simulink model "MotorTests"  (R2023b)
settings: Solver=VariableStepAuto  StartTime=0.0  StopTime=10.0  RelTol=1e-3
libraries: spsCurrentMeasurementLib x4, spsVoltageMeasurementLib x4, spsGroundLib x3, spsAsynchronousMachineSIUnitsLib x2, spsRMSLib x2, spspowerguiLib x2, mcbacimparamestlib x2, spsDCVoltageSourceLib x1, spsPowerPositiveSequenceLib x1, spsThreePhaseProgrammableVoltageSourceLib x1
settings Model: Creator=Jakob  LastModifiedBy=Jakob

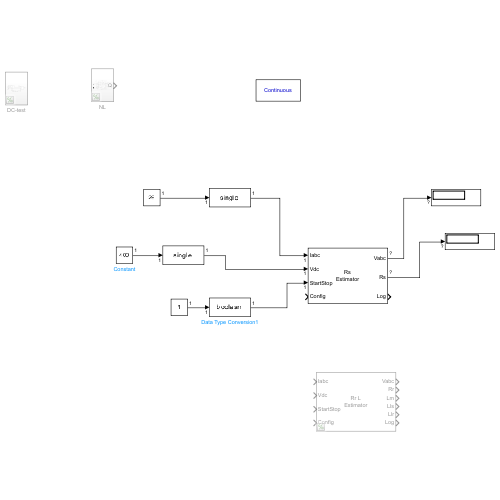
[thumbnail: Simulink's stored preview of the top-level diagram]
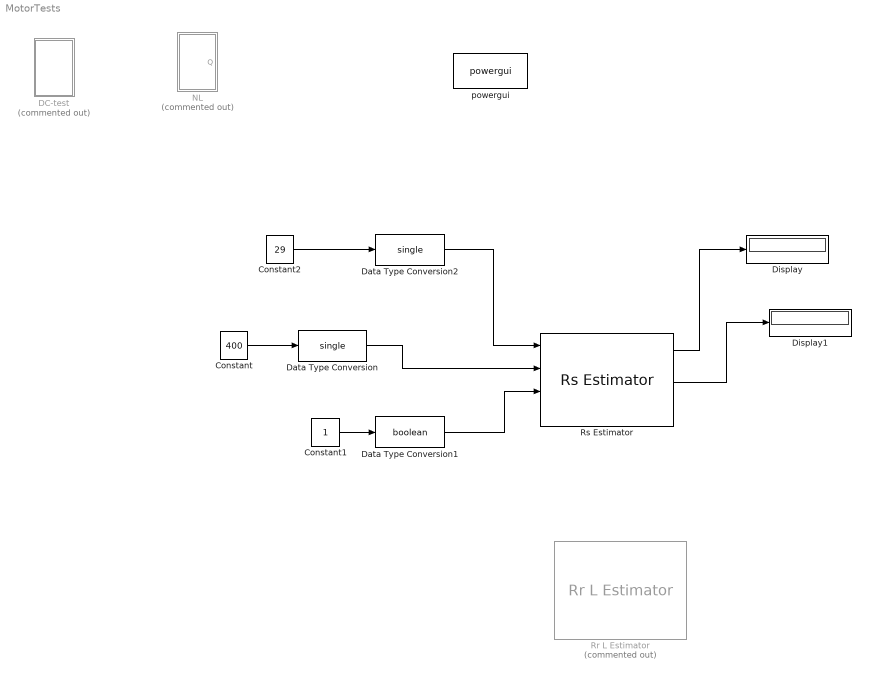
== system MotorTests ==
  Constant : Constant  Value=400
  Constant1 : Constant
  Constant2 : Constant  Value=29
  DC-test : Subsystem  Commented=on
  Data Type Conversion : DataTypeConversion  OutDataTypeStr=single  SaturateOnIntegerOverflow=off  RndMeth=Floor
  Data Type Conversion1 : DataTypeConversion  OutDataTypeStr=boolean  SaturateOnIntegerOverflow=off  RndMeth=Floor
  Data Type Conversion2 : DataTypeConversion  OutDataTypeStr=single  SaturateOnIntegerOverflow=off  RndMeth=Floor
  Display : Display
  Display1 : Display
  NL : Subsystem  Commented=on
  Rr L Estimator : mcbacimparamestlib/Rr L Estimator  Commented=on
      settings: LibrarySourceBlock=mcblib/Parameter Estimation/ACIM Parameter Estimation/Rr L Estimator
  Rs Estimator : mcbacimparamestlib/Rs Estimator
      settings: LibrarySourceBlock=mcblib/Parameter Estimation/ACIM Parameter Estimation/Rs Estimator
  powergui : spspowerguiLib/powergui  Priority=1  SimulationMode=Continuous  SampleTime=50e-6  frequency=60  Iterations=50  frequencyindice=50  Pbase=100e6  ErrMax=1e-4  UnitsV=kV  UnitsW=MW  buscounter=0  FunctionMessages=off  echomessages=off  EnableUseOfTLC=off  CurrentSourceSwitches=off  DisableSnubberDevices=off  DisableRonSwitches=off  DisableVfSwitches=off  DisplayEquations=off  AutomaticDiscreteSolvers=off  SolverType=Tustin/Backward Euler (TBE)  Interpol=off  ExternalGateDelay=off  methode=off  Ts=100  x0status=blocks  SPID=on  SwTol=0  HookPort=off  NonlinearTolerance=1e-4  nMaxIteration=100  ContinueOnMaxIteration=off  RestoreLinks=warning  ResistiveCurrentMeasurement=off  Frange=[0:2:500]  Ylog=off  Xlog=on  ShowGrid=off  save=off  variable=ZData  structure=0  ZoomFFT=off  StartTime=0.0  cycles=1  DisplayStyle=1  fundamental=60  FreqAxis=off  MaxFrequency=1000  frequencyindicesteady=1  RmsSteady=1  display=off
  wires:
  Constant/1 -> Data Type Conversion/1
  Constant1/1 -> Data Type Conversion1/1
  Rs Estimator/1 -> Display/1
  Rs Estimator/2 -> Display1/1
  Data Type Conversion/1 -> Rs Estimator/2
  Data Type Conversion1/1 -> Rs Estimator/3
  Constant2/1 -> Data Type Conversion2/1
  Data Type Conversion2/1 -> Rs Estimator/1

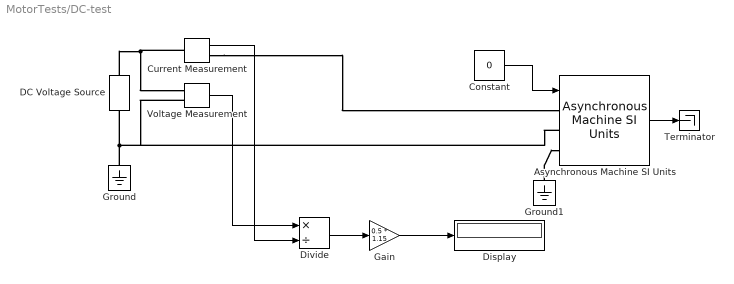
== system MotorTests/DC-test ==
  Asynchronous Machine SI Units : spsAsynchronousMachineSIUnitsLib/Asynchronous Machine SI Units  RotorType=Double squirrel-cage  PresetModel=No  MechanicalLoad=Torque Tm  ShowDetailedParameters=on  ReferenceFrame=Rotor  Units=SI  MeasurementBus=off  NominalParameters=[1.5e+04 400 50]  VoltageRatio=1  Stator=[0.619 0.0005084]  Rotor=[0.6258 0.005473]  Cage1=[0.2781 0.002617]  Cage2=[0.5433 0.0005084]  Lm=0.04417  Mechanical=[0.13 0.005879 2]  PolePairs=2  InitialConditions=[0 0 0 0 0 0 0 0]  SimulateSaturation=off  Saturation=[14.03593122, 27.81365428, 53.79336849, 72.68890987, 97.98006896, 148.6815601, 215.7428561, 302.9841135, 428.7778367 ; 230, 322, 414, 460, 506, 552, 598, 644, 690]  LoadFlowParameters=1492000  TsPowergui=0  TsBlock=-1  IterativeModel=Trapezoidal non iterative  IterativeDiscreteModel=Trapezoidal non iterative  Pmec=1.492e+006
  Constant : Constant  Value=0
  Current Measurement : spsCurrentMeasurementLib/Current Measurement  PhasorSimulation=off  OutputType=Complex  PSBequivalent=0
  DC Voltage Source : spsDCVoltageSourceLib/DC Voltage Source  Amplitude=9  Measurements=None
  Display : Display
  Divide : Product  Inputs=*/
  Gain : Gain  Gain=0.5 * 1.15
  Ground : spsGroundLib/Ground  LConnTagsString=a
  Ground1 : spsGroundLib/Ground  LConnTagsString=a
  Terminator : Terminator
  Voltage Measurement : spsVoltageMeasurementLib/Voltage Measurement  PhasorSimulation=off  OutputType=Complex  PSBequivalent=0
  wires:
  Constant/1 -> Asynchronous Machine SI Units/1
  Voltage Measurement/1 -> Divide/1
  Divide/1 -> Gain/1
  Asynchronous Machine SI Units/1 -> Terminator/1
  Gain/1 -> Display/1
  Current Measurement/1 -> Divide/2
  connections:
  Ground1/LConn1 -- Asynchronous Machine SI Units/LConn3
  DC Voltage Source/RConn1 -- Voltage Measurement/LConn1 -- Current Measurement/LConn1
  Ground/LConn1 -- Asynchronous Machine SI Units/LConn2 -- Voltage Measurement/LConn2 -- DC Voltage Source/LConn1
  Current Measurement/RConn1 -- Asynchronous Machine SI Units/LConn1

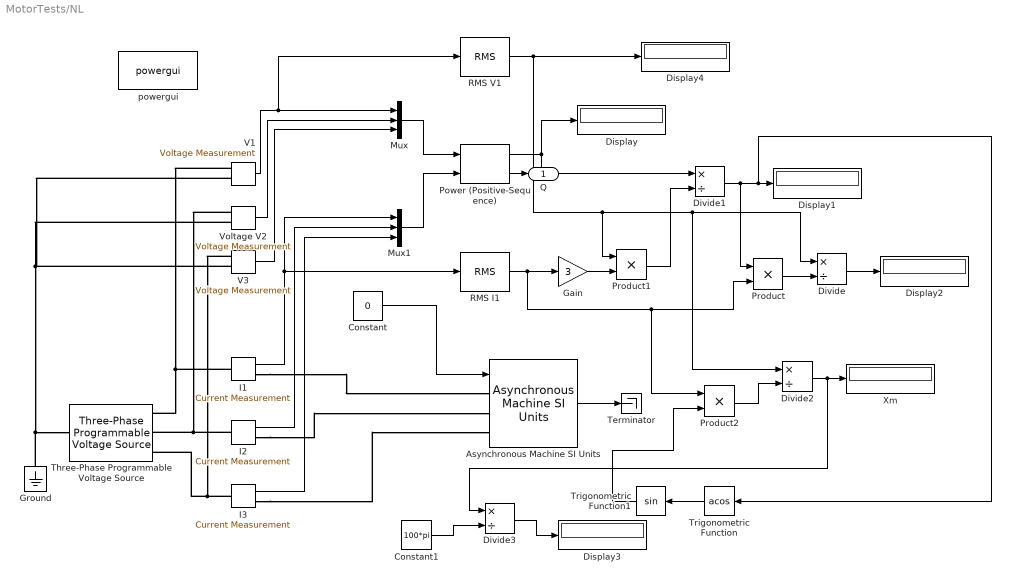
== system MotorTests/NL ==
  Asynchronous Machine SI Units : spsAsynchronousMachineSIUnitsLib/Asynchronous Machine SI Units  RotorType=Double squirrel-cage  PresetModel=No  MechanicalLoad=Torque Tm  ShowDetailedParameters=on  ReferenceFrame=Rotor  Units=SI  MeasurementBus=off  NominalParameters=[1.5e+04 400 50]  VoltageRatio=1  Stator=[0.619 0.0005084]  Rotor=[0.6258 0.005473]  Cage1=[0.2781 0.002617]  Cage2=[0.5433 0.0005084]  Lm=0.04417  Mechanical=[0.13 0.005879 2]  PolePairs=2  InitialConditions=[1 0 0 0 0 0 0 0]  SimulateSaturation=off  Saturation=[14.03593122, 27.81365428, 53.79336849, 72.68890987, 97.98006896, 148.6815601, 215.7428561, 302.9841135, 428.7778367 ; 230, 322, 414, 460, 506, 552, 598, 644, 690]  LoadFlowParameters=1492000  TsPowergui=0  TsBlock=-1  IterativeModel=Trapezoidal non iterative  IterativeDiscreteModel=Trapezoidal non iterative  Pmec=1.492e+006
  Constant : Constant  Value=0
  Constant1 : Constant  Value=100*pi
  Display{,1..4} (5 alike) : Display
  Divide{,1..3} (4 alike) : Product  Inputs=*/
  Gain : Gain  Gain=3
  Ground : spsGroundLib/Ground  LConnTagsString=a
  I1 : spsCurrentMeasurementLib/Current Measurement  PhasorSimulation=off  OutputType=Complex  PSBequivalent=0
  I2 : spsCurrentMeasurementLib/Current Measurement  PhasorSimulation=off  OutputType=Complex  PSBequivalent=0
  I3 : spsCurrentMeasurementLib/Current Measurement  PhasorSimulation=off  OutputType=Complex  PSBequivalent=0
  Mux : Mux  Inputs=3
  Mux1 : Mux  Inputs=3
  Power (Positive-Sequence) : spsPowerPositiveSequenceLib/Power (Positive-Sequence)  Freq=60  Vinit=[0, 0]  Iinit=[0, 0]  Ts=0
      settings: LibrarySourceBlock=|
      | sps_lib/Sensors and Measurements/Power
      | (Positive-Sequence)
  Product : Product
  Product1 : Product
  Product2 : Product
  RMS I1 : spsRMSLib/RMS  TrueRMS=on  Freq=60  RMSInit=120  Ts=0
  RMS V1 : spsRMSLib/RMS  TrueRMS=on  Freq=60  RMSInit=120  Ts=0
  Terminator : Terminator
  Three-Phase Programmable Voltage Source : spsThreePhaseProgrammableVoltageSourceLib/Three-Phase Programmable Voltage Source  PositiveSequence="[400  0 50]"  VariationEntity=None  VariationType=Table of time-amplitude pairs  VariationTypeAlt=Step  VariationStep=0.5  VariationRate=10  VariationMagnitude=0.3  VariationFrequency=2  VariationTiming=[1 2]  VariationPhaseA=off  Amplitudes=[1 0.8 1.2 1.0]  TimeValues=[0 0.1 0.15 0.2]  HarmonicGeneration=off  HarmonicA=[3 0.2 -25 0]  HarmonicB=[2 0.15 35 2]  Timing="[0.05  3]"  BusType=swing  Pref=0  Qref=0  Qmin=-inf  Qmax=inf
  Trigonometric Function : Trigonometry  Operator=acos
  Trigonometric Function1 : Trigonometry
  V1 : spsVoltageMeasurementLib/Voltage Measurement  PhasorSimulation=off  OutputType=Complex  PSBequivalent=0
  V3 : spsVoltageMeasurementLib/Voltage Measurement  PhasorSimulation=off  OutputType=Complex  PSBequivalent=0
  Voltage V2 : spsVoltageMeasurementLib/Voltage Measurement  PhasorSimulation=off  OutputType=Complex  PSBequivalent=0
  Xm : Display
  powergui : spspowerguiLib/powergui  Priority=1  SimulationMode=Continuous  SampleTime=50e-6  frequency=60  Iterations=50  frequencyindice=50  Pbase=100e6  ErrMax=1e-4  UnitsV=kV  UnitsW=MW  buscounter=0  FunctionMessages=off  echomessages=off  EnableUseOfTLC=off  CurrentSourceSwitches=off  DisableSnubberDevices=off  DisableRonSwitches=off  DisableVfSwitches=off  DisplayEquations=off  AutomaticDiscreteSolvers=off  SolverType=Tustin/Backward Euler (TBE)  Interpol=off  ExternalGateDelay=off  methode=off  Ts=100  x0status=blocks  SPID=on  SwTol=0  HookPort=off  NonlinearTolerance=1e-4  nMaxIteration=100  ContinueOnMaxIteration=off  RestoreLinks=warning  ResistiveCurrentMeasurement=off  Frange=[0:2:500]  Ylog=off  Xlog=on  ShowGrid=off  save=off  variable=ZData  structure=0  ZoomFFT=off  StartTime=0.0  cycles=1  DisplayStyle=1  fundamental=60  FreqAxis=off  MaxFrequency=1000  frequencyindicesteady=1  RmsSteady=1  display=off
  Q : Outport
  wires:
  RMS V1/1 -> Display4/1, Divide2/1, Divide/1, Product1/1
  Constant1/1 -> Divide3/2
  I1/1 -> RMS I1/1, Mux1/1
  Divide/1 -> Display2/1
  Mux1/1 -> Power (Positive-Sequence)/2
  V1/1 -> RMS V1/1, Mux/1
  I3/1 -> Mux1/3
  Power (Positive-Sequence)/1 -> Divide1/1, Display/1
  Constant/1 -> Asynchronous Machine SI Units/1
  Mux/1 -> Power (Positive-Sequence)/1
  RMS I1/1 -> Product2/1, Product/2, Gain/1
  Product/1 -> Divide/2
  Divide2/1 -> Divide3/1, Xm/1
  Asynchronous Machine SI Units/1 -> Terminator/1
  Divide1/1 -> Product/1, Display1/1, Trigonometric Function/1
  Trigonometric Function/1 -> Trigonometric Function1/1
  Gain/1 -> Product1/2
  Product1/1 -> Divide1/2
  Power (Positive-Sequence)/2 -> Q/1
  Voltage V2/1 -> Mux/2
  Product2/1 -> Divide2/2
  V3/1 -> Mux/3
  I2/1 -> Mux1/2
  Trigonometric Function1/1 -> Product2/2
  Divide3/1 -> Display3/1
  connections:
  I3/LConn1 -- V3/LConn1 -- Three-Phase Programmable Voltage Source/RConn3
  Ground/LConn1 -- V1/LConn2 -- Voltage V2/LConn2 -- V3/LConn2 -- Three-Phase Programmable Voltage Source/LConn1
  I3/RConn1 -- Asynchronous Machine SI Units/LConn3
  I1/RConn1 -- Asynchronous Machine SI Units/LConn1
  I2/RConn1 -- Asynchronous Machine SI Units/LConn2
  I2/LConn1 -- Voltage V2/LConn1 -- Three-Phase Programmable Voltage Source/RConn2
  I1/LConn1 -- V1/LConn1 -- Three-Phase Programmable Voltage Source/RConn1
